simulink model "DTMF_Telefonie_Project_Crehul_Hornai"  (R2018b)
settings: Solver=VariableStepAuto  StartTime=0.0  StopTime=100  RelTol=1e-3
undefined symbols (not defined in the file): fdesignblkfcn, gcbh
libraries: simulink x12, dspfdesign x7
(part 3 of 4)

== system DTMF_Telefonie_Project_Crehul_Hornai/DTMF Detector and Decoder/Subsystem1/770Hz Bandpass Filter ==
  In : Inport
  Generated Filter Block : DiscreteFir  Tag=BlockMethodSubSystem  Coefficients=[-0.00115171448739976841 -6.2045649466851982e-05 -3.2139792056238561e-05 1.09463265911958867e-05 5.97085892407322755e-05 0.000100709352649991498 0.000126161821806573598 0.000127231537284110217 0.000104894657608967405 6.10750914818174086e-05 7.46695113397520885e-06 -4.62497542373604444e-05 -8.47798084930044202e-05 -0.000101054989633250943 -8.68894767499833916e-05 -4.91119865411407831e-05 5.4099761280029194e-06 6.74173823690992283e-05 0.000119260925398808086 0.000149611402815285266 0.000150867245733493074 0.000120958574369038879 6.68104026648620036e-05 -8.3979354246251775e-07 -6.53351250350642492e-05 -0.000112859248145101131 -0.000130455323326076657 -0.000114806989127967966 -6.71321220113085208e-05 7.12581153046410939e-07 7.57898909437479656e-05 0.000138024851659114805 0.000174352723502319918 0.000174710937480642824 0.000138593908123871897 7.26851250080165923e-05 -7.41690532358747073e-06 -8.45549315840361804e-05 -0.000139549697866669063 -0.000160366739214787149 -0.00014009778440222595 -8.38111108748265058e-05 -2.44451318231835545e-06 8.41503440451062731e-05 0.000157165582713895491 0.000197857611481149203 0.000197946140746531026 0.000154448841019343532 7.84135135782778291e-05 -1.46257209000613154e-05 -0.000102141166355649562 -0.000164997889975689559 -0.00018686206401534065 -0.000163242311520504346 -9.75229357316404529e-05 -5.64034899509552497e-06 9.27985535325293303e-05 0.000173694984794322323 0.000219383097775983785 0.000217334944960366917 0.000168488240410150179 8.2093757929535419e-05 -2.07883010015774954e-05 -0.000118363297804733366 -0.000186252046200404428 -0.000209928845013323271 -0.000181905281352516372 -0.00010950413722201984 -7.56589274818067828e-06 9.92372049102201517e-05 0.000187650923866160583 0.000235586346351471026 0.000232865943559337285 0.000178182685500632423 8.50901343910520115e-05 -2.66061096263520321e-05 -0.000130028906414838066 -0.000202526922996726757 -0.00022568410271670762 -0.000195411317069056492 -0.000116766425967328386 -9.16438973955950933e-06 0.000104207454859655841 0.000195701281425481391 0.000245511198747249576 0.000240484481621172749 0.000183009228164836887 8.47227045778771275e-05 -3.04441693818940581e-05 -0.000137445188713204713 -0.00021017663912385352 -0.000233229871489936584 -0.000200001752738408495 -0.00011943596847820365 -8.75413017988957778e-06 0.000105041419590837281 0.000197209243667155953 0.000245083036854206208 0.000239235391780027659 0.000179724536784867019 8.18716508768826262e-05 -3.31204208596507128e-05 -0.000137298758944944758 -0.000208223498353422333 -0.000228427211619664948 -0.000195112000448446942 -0.000114926121635641233 -8.10993716863226202e-06 0.000101850516821929337 0.000188388973889463268 0.000233234276234002818 0.000225211498952974758 0.000168219453055813185 7.4558582370404464e-05 -3.2368079983214346e-05 -0.000129272279857957058 -0.000192736463926152695 -0.000210248558618575995 -0.000177261505807543157 -0.000103720323264914257 -5.92329729190346072e-06 9.17858153168062997e-05 0.000168489960018308521 0.000205750488927836138 0.000197366009839074468 0.00014517004247161262 6.36256431443505896e-05 -2.90927482831460429e-05 -0.000110133157340498375 -0.000162747944417547833 -0.000174576796784631618 -0.000145772733770913997 -8.3139568878139343e-05 -3.71954468539239386e-06 7.49864329870016978e-05 0.000133703943476896642 0.000161301808092614071 0.000151647449644298988 0.000110292844954072971 4.706971959873049e-05 -2.09947868436491381e-05 -7.93513307059707119e-05 -0.000114040879135501524 -0.000120064191715578547 -9.69049730280406064e-05 -5.34783642157470041e-05 -2.06189326351679039e-07 4.8478329733259596e-05 8.30289957149718105e-05 9.56081930328673158e-05 8.69759271064881375e-05 6.04574854350258158e-05 2.5861265825665369e-05 -8.68259134646776065e-06 -3.35573183046643415e-05 -4.55081387884723448e-05 -4.27141974058827759e-05 -3.01259267542505847e-05 -1.23495985288062018e-05 2.88279091327676984e-06 1.2274610911791042e-05 1.28199961432636476e-05 7.66025856037454503e-06 -2.36701549149315182e-07 ...(+19709 chars)]  InputProcessing=Columns as channels (frame based)
  Out : Outport
  wires:
  In/1 -> Generated Filter Block/1
  Generated Filter Block/1 -> Out/1

== system DTMF_Telefonie_Project_Crehul_Hornai/DTMF Detector and Decoder/Subsystem1/852Hz Bandpass Filter ==
  In : Inport
  Generated Filter Block : DiscreteFir  Tag=BlockMethodSubSystem  Coefficients=[-0.000259867897103560001 -0.000252995169651927326 0.000395067000004355434 -0.000155035857658841525 -5.88620733905397458e-05 -0.00023179640334809745 -0.000182829742796099281 -0.000166980085288837167 -6.97860028735931809e-05 2.05130585547824233e-05 0.000114335533241517764 0.000171595157908201976 0.000185980566935853167 0.000147691328940777671 6.69484864525067992e-05 -3.79938069153539049e-05 -0.000138932721342923087 -0.000207569103719058926 -0.000221560153518105251 -0.000172450870124806019 -6.88832378688698218e-05 6.38553282803985426e-05 0.000189753453509081441 0.000271403812019560455 0.000280936608477930499 0.000209063658943275894 6.9592520523719512e-05 -0.000102581926456920105 -0.000259793969267451265 -0.000354641223950492857 -0.000353918405510016511 -0.000249710338059728207 -6.38455814969149469e-05 0.000156012953423071744 0.000348306539322294447 0.000454534291244017329 0.000436793018923241328 0.000290475016776262725 4.83311336538223119e-05 -0.000226371375925976334 -0.000455985042686667575 -0.000570246702743955423 -0.000527371727264558257 -0.000328403362491726583 -1.9967993565558461e-05 0.00031602529553136072 0.000583945878882551257 0.000701269142239906076 0.00062372614868338506 0.000360566975427972542 -2.42385931337404778e-05 -0.000427321569414288978 -0.000733109700209630421 -0.000846917903208209378 -0.000723578252331691244 -0.000383926743315451545 8.73969799036579192e-05 0.000562398687364638276 0.000904192578562196801 0.00100595087473387738 0.000824245702745070937 0.000395106827790690969 -0.000172369712824167141 -0.000723265620829646435 -0.00109740196380214748 -0.00117664464885476865 -0.000922587748817896899 -0.000390544604431714037 0.000282731389067540813 0.000911267170375920079 0.00131144838963140006 0.00135687742245041258 0.00101599855371768731 0.000366089453151203245 -0.000421289549147785334 -0.00112742370990784476 -0.00154637677024365978 -0.001543305429094848 -0.00109873620738014724 -0.000318950110548274718 0.000589698021381435621 0.00137255877670164903 0.0017998583504240627 0.00173316359474022215 0.00116812008921605027 0.000244165437324022608 -0.000790808500201104435 -0.00164643042899360534 -0.00206961892334233408 -0.00192133226394149907 -0.00121887581074967715 -0.000138847257337018035 0.00102604700820171425 0.00194774090263288261 0.00235270044054247717 0.00210434025977529211 0.00124704116327450064 -2.58764053679085841e-09 -0.00129631791216740233 -0.00227512700389562259 -0.00264488063136342514 -0.00227658320224804166 -0.00124719413458679687 0.00017603693854455107 0.00160223473537411763 0.00262627986742082573 0.00294182650027749199 0.00243323486014204293 0.00121572663489594537 -0.000390611172753166879 -0.00194232660981847184 -0.0029973281757985676 -0.00323815614798470507 -0.00256877675281262435 -0.00114824471483653619 0.000645636479673961355 0.00231573057011790883 0.00338456526980192686 0.0035286335246959618 0.0026776475037035446 0.00104084949894931236 -0.000942302025141843473 -0.00272037565042822704 -0.00378333884022261872 -0.00380732057345092509 -0.00275460294378229026 -0.000890498067367577538 0.00128021083410175484 0.00315284077961586759 0.00418761628573812578 0.0040679646320084719 0.00279429876515000517 0.00069524696044065892 -0.00165878503537046293 -0.0036085241518536669 -0.00459150842273998126 -0.00430369705723419871 -0.00279251568861569981 -0.000452904519039117092 0.00207552627682001858 0.00408265433720936873 0.00498840057340856936 0.00450863263314901612 0.00274463782156249454 0.000162741324454134803 -0.00252752059862553511 -0.00456959102454090275 -0.00537093539610358165 -0.00467663485667387142 -0.00264739494962847174 0.000174572050301093757 0.00301126727079113537 0.00506244961295426905 0.00573245317874398076 0.00480164109961274573 0.0024981860400853451 -0.0005580444799926647 -0.0035212732157224977 -0.00555440146680824792 -0.00606514735407167379 -0.00487884534940971441 -0.00229532723572540903 0.00098497420004075068 0.0040519710704794154 0.00603762662801356903 0.00636229767258047595 0.00490325416211494312 ...(+7764 chars)]  InputProcessing=Columns as channels (frame based)
  Out : Outport
  wires:
  In/1 -> Generated Filter Block/1
  Generated Filter Block/1 -> Out/1
